simulink model "Quadrotor_Controller"  (R2019a)
settings: Solver=ode14x  StartTime=0.0  StopTime=10  FixedStep=1/100  RelTol=1e-3  EnableMultiTasking=on
undefined symbols (not defined in the file): Ap, cd, dfod, DiscIntNeverNeededParam, ioKd, ioKi, ioKp, Kd, Kp, kt, L, Newton, Pitch_0, Raphson, rho, Roll_0, Rp, X, Y, Z
libraries: sm_lib x122, fl_ps_legacy_lib x41, fl_lib x28, nesl_utility x14, sharedtransform x12, simulink x5, Electrical_Library x4, Mechanical_Library x4
(part 4 of 5)

== system Quadrotor_Controller/Quadrotor Mechanics/HUB_1_RIGID ==
  ReferenceFrame : sm_lib/Frames and Transforms/Reference Frame
  Solid : sm_lib/Body Elements/Solid  InertiaType=Custom  Mass=0.0035073100000000005  MassUnits=kg  CenterOfMass=[0.0036894251968503933 0.014803307086614171 -0.020664488188976374]  CenterOfMassUnits=in  MomentsOfInertia=[0.001075372000744001 0.0010304544609089214 0.0019974579949159888]  MomentsOfInertiaUnits=kg*in^2  ProductsOfInertia=[-1.7442184884369763e-05 2.6471572943145881e-07 3.2888585777171548e-06]  ProductsOfInertiaUnits=kg*in^2  BasedOnType=Density  Density=1000  DensityUnits=kg/(m^3)  DoExposeReferenceFrame=on  SerializedFrames=<Frames/>  GraphicType=FromGeometry  MarkerShape=Sphere  MarkerSize=10  MarkerSizeUnits=m  GraphicVisPropType=SimpleVisualProperties  GraphicDiffuseColor=[0.792157 0.819608 0.933333]  GraphicSpecularColor=[0.5 0.5 0.5 1.0]  GraphicAmbientColor=[0.15 0.15 0.15 1.0]  GraphicEmissiveColor=[0.0 0.0 0.0 1.0]  GraphicShininess=75  GraphicOpacity=1  GeometryShape=FromFile  RectangleSize=[1 1]  RectangleSizeUnits=m  BrickDimensions=[1 1 1]  BrickDimensionUnits=m  CylinderRadius=1  CylinderRadiusUnits=m  CylinderLength=1  CylinderLengthUnits=m  SphereRadius=1  SphereRadiusUnits=m  EllipsoidRadii=[1 1 1]  EllipsoidRadiiUnits=m  ExtrusionCrossSection=[1 1; -1 1; -1 -1; 1 -1]  ExtrusionCrossSectionUnits=m  ExtrusionLength=1  ExtrusionLengthUnits=m  PolygonNumSides=3  PolygonOuterRadius=1  PolygonOuterRadiusUnits=m  ExtGeomFileType=STL  ExtGeomFileName=HUB_Default_sldprt.STL  ExtGeomFileUnits=in  RevolutionCrossSection=[1 1; 1 -1; 2 -1; 2 1]  RevolutionCrossSectionUnits=m  RevolutionExtent=Full  RevolutionAngle=180  RevolutionAngleUnits=deg
  F : PMIOPort  Side=Left
  connections:
  Solid/RConn1 -- ReferenceFrame/RConn1 -- F/RConn1

== system Quadrotor_Controller/Subsystem/Triggered Subsystem ==
  In1 : Inport
  Trigger : TriggerPort  VariantControl=Variant
  Out1 : Outport
  wires:
  In1/1 -> Out1/1

== system Quadrotor_Controller/Controller/FOPD/Fractional DD ==
  In1 : Inport
  Discrete Transfer Fcn : DiscreteTransferFcn  Commented=on  Numerator=num  Denominator=den  SampleTime=Ts
  Rate Transition : RateTransition  OutPortSampleTime=Ts
  Rate Transition1 : RateTransition  OutPortSampleTime=0.01
  Transfer Fcn : TransferFcn  Numerator=num  Denominator=den
  Out1 : Outport
  wires:
  Transfer Fcn/1 -> Rate Transition1/1
  In1/1 -> Rate Transition/1
  Rate Transition/1 -> Transfer Fcn/1
  Rate Transition1/1 -> Out1/1

== system Quadrotor_Controller/Controller/FOPD GNCC IRID/Fractional DD ==
  In1 : Inport
  Discrete Transfer Fcn : DiscreteTransferFcn  Commented=on  Numerator=num  Denominator=den  SampleTime=Ts
  Rate Transition : RateTransition  OutPortSampleTime=Ts
  Rate Transition1 : RateTransition  OutPortSampleTime=0.01
  Transfer Fcn : TransferFcn  Numerator=num  Denominator=den
  Out1 : Outport
  wires:
  Transfer Fcn/1 -> Rate Transition1/1
  In1/1 -> Rate Transition/1
  Rate Transition/1 -> Transfer Fcn/1
  Rate Transition1/1 -> Out1/1

== system Quadrotor_Controller/Controller/FOPI- GNCC IRID/Fractional DD ==
  In1 : Inport
  Discrete Transfer Fcn : DiscreteTransferFcn  Commented=on  Numerator=num  Denominator=den  SampleTime=Ts
  Rate Transition : RateTransition  OutPortSampleTime=Ts
  Rate Transition1 : RateTransition  OutPortSampleTime=0.01
  Transfer Fcn : TransferFcn  Numerator=num  Denominator=den
  Out1 : Outport
  wires:
  Transfer Fcn/1 -> Rate Transition1/1
  In1/1 -> Rate Transition/1
  Rate Transition/1 -> Transfer Fcn/1
  Rate Transition1/1 -> Out1/1

== system Quadrotor_Controller/Controller/FOPID/Fractional DD ==
  In1 : Inport
  Discrete Transfer Fcn : DiscreteTransferFcn  Commented=on  Numerator=num  Denominator=den  SampleTime=Ts
  Rate Transition : RateTransition  OutPortSampleTime=Ts
  Rate Transition1 : RateTransition  OutPortSampleTime=0.01
  Transfer Fcn : TransferFcn  Numerator=num  Denominator=den
  Out1 : Outport
  wires:
  Transfer Fcn/1 -> Rate Transition1/1
  In1/1 -> Rate Transition/1
  Rate Transition/1 -> Transfer Fcn/1
  Rate Transition1/1 -> Out1/1

== system Quadrotor_Controller/Controller/FOPID/Fractional DD1 ==
  In1 : Inport
  Discrete Transfer Fcn : DiscreteTransferFcn  Commented=on  Numerator=num  Denominator=den  SampleTime=Ts
  Rate Transition : RateTransition  OutPortSampleTime=Ts
  Rate Transition1 : RateTransition  OutPortSampleTime=0.01
  Transfer Fcn : TransferFcn  Numerator=num  Denominator=den
  Out1 : Outport
  wires:
  Transfer Fcn/1 -> Rate Transition1/1
  In1/1 -> Rate Transition/1
  Rate Transition/1 -> Transfer Fcn/1
  Rate Transition1/1 -> Out1/1

== system Quadrotor_Controller/Ground Stop/FloorStop1/Translational Simscape Intf1 ==
  Ideal Force Sensor : fl_lib/Mechanical/Mechanical Sensors/Ideal Force Sensor
  Ideal Translational Velocity Source : fl_lib/Mechanical/Mechanical Sources/Ideal Translational Velocity Source
  V : PMIOPort  Side=Left
  F : PMIOPort  Port=2  Side=Right
  R : PMIOPort  Port=3  Side=Left
  C : PMIOPort  Port=4  Side=Right
  connections:
  V/RConn1 -- Ideal Translational Velocity Source/RConn1
  F/RConn1 -- Ideal Force Sensor/RConn2
  Ideal Force Sensor/LConn1 -- Ideal Translational Velocity Source/RConn2
  R/RConn1 -- Ideal Translational Velocity Source/LConn1
  Ideal Force Sensor/RConn1 -- C/RConn1

== system Quadrotor_Controller/Ground Stop/FloorStop2/Translational Simscape Intf1 ==
  Ideal Force Sensor : fl_lib/Mechanical/Mechanical Sensors/Ideal Force Sensor
  Ideal Translational Velocity Source : fl_lib/Mechanical/Mechanical Sources/Ideal Translational Velocity Source
  V : PMIOPort  Side=Left
  F : PMIOPort  Port=2  Side=Right
  R : PMIOPort  Port=3  Side=Left
  C : PMIOPort  Port=4  Side=Right
  connections:
  Ideal Force Sensor/RConn1 -- C/RConn1
  R/RConn1 -- Ideal Translational Velocity Source/LConn1
  Ideal Force Sensor/LConn1 -- Ideal Translational Velocity Source/RConn2
  F/RConn1 -- Ideal Force Sensor/RConn2
  V/RConn1 -- Ideal Translational Velocity Source/RConn1

== system Quadrotor_Controller/Ground Stop/FloorStop3/Translational Simscape Intf1 ==
  Ideal Force Sensor : fl_lib/Mechanical/Mechanical Sensors/Ideal Force Sensor
  Ideal Translational Velocity Source : fl_lib/Mechanical/Mechanical Sources/Ideal Translational Velocity Source
  V : PMIOPort  Side=Left
  F : PMIOPort  Port=2  Side=Right
  R : PMIOPort  Port=3  Side=Left
  C : PMIOPort  Port=4  Side=Right
  connections:
  Ideal Force Sensor/RConn1 -- C/RConn1
  R/RConn1 -- Ideal Translational Velocity Source/LConn1
  Ideal Force Sensor/LConn1 -- Ideal Translational Velocity Source/RConn2
  F/RConn1 -- Ideal Force Sensor/RConn2
  V/RConn1 -- Ideal Translational Velocity Source/RConn1

== system Quadrotor_Controller/Ground Stop/FloorStop4/Translational Simscape Intf1 ==
  Ideal Force Sensor : fl_lib/Mechanical/Mechanical Sensors/Ideal Force Sensor
  Ideal Translational Velocity Source : fl_lib/Mechanical/Mechanical Sources/Ideal Translational Velocity Source
  V : PMIOPort  Side=Left
  F : PMIOPort  Port=2  Side=Right
  R : PMIOPort  Port=3  Side=Left
  C : PMIOPort  Port=4  Side=Right
  connections:
  Ideal Force Sensor/RConn1 -- C/RConn1
  R/RConn1 -- Ideal Translational Velocity Source/LConn1
  Ideal Force Sensor/LConn1 -- Ideal Translational Velocity Source/RConn2
  F/RConn1 -- Ideal Force Sensor/RConn2
  V/RConn1 -- Ideal Translational Velocity Source/RConn1

== system Quadrotor_Controller/Measurements/Bus Mapping/Subsystem ==
  DCM : Inport
  AxisRotDefault : sharedtransform/Direction Cosine Matrix to Rotation Angles/AxisRotDefault  SystemSampleTime=-1
      settings: SourceProductName=Aerospace Blockset  SourceProductBaseCode=AE
  AxisRotZeroR3 : sharedtransform/Direction Cosine Matrix to Rotation Angles/AxisRotZeroR3  SystemSampleTime=-1
      settings: SourceProductName=Aerospace Blockset  SourceProductBaseCode=AE
  Get DCM Values : sharedtransform/Direction Cosine Matrix to Rotation Angles/Get DCM Values  SystemSampleTime=-1
      settings: SourceProductName=Aerospace Blockset  SourceProductBaseCode=AE
  If : If  IfExpression=(u1>=1)|(u1<=-1)
  Merge : Merge
  Selector4 : Selector  InputPortWidth=7  IndexOptions=Index vector (dialog)  Indices=3  OutputSizes=1
  Out1 : Outport
  wires:
  Merge/1 -> Out1/1
  If/1 -> AxisRotZeroR3/Action
  Selector4/1 -> If/1  "r21"
  DCM/1 -> Get DCM Values/1
  Get DCM Values/1 -> Selector4/1, AxisRotZeroR3/1, AxisRotDefault/1
  AxisRotDefault/1 -> Merge/2
  AxisRotZeroR3/1 -> Merge/1
  If/2 -> AxisRotDefault/Action

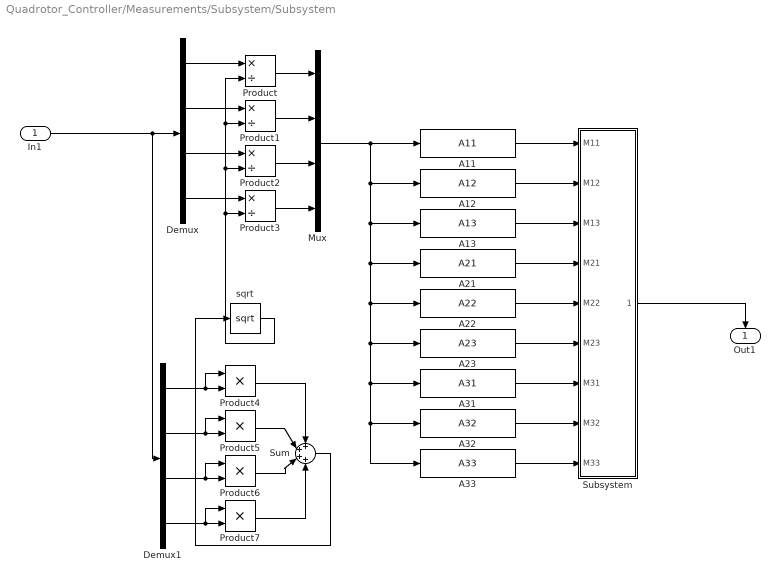
== system Quadrotor_Controller/Measurements/Subsystem/Subsystem ==
  In1 : Inport
  A11 : sharedtransform/Quaternions to  Direction Cosine Matrix/A11  SystemSampleTime=-1
      settings: SourceProductName=Aerospace Blockset  SourceProductBaseCode=AE
  A12 : sharedtransform/Quaternions to  Direction Cosine Matrix/A12  SystemSampleTime=-1
      settings: SourceProductName=Aerospace Blockset  SourceProductBaseCode=AE
  A13 : sharedtransform/Quaternions to  Direction Cosine Matrix/A13  SystemSampleTime=-1
      settings: SourceProductName=Aerospace Blockset  SourceProductBaseCode=AE
  A21 : sharedtransform/Quaternions to  Direction Cosine Matrix/A21  SystemSampleTime=-1
      settings: SourceProductName=Aerospace Blockset  SourceProductBaseCode=AE
  A22 : sharedtransform/Quaternions to  Direction Cosine Matrix/A22  SystemSampleTime=-1
      settings: SourceProductName=Aerospace Blockset  SourceProductBaseCode=AE
  A23 : sharedtransform/Quaternions to  Direction Cosine Matrix/A23  SystemSampleTime=-1
      settings: SourceProductName=Aerospace Blockset  SourceProductBaseCode=AE
  A31 : sharedtransform/Quaternions to  Direction Cosine Matrix/A31  SystemSampleTime=-1
      settings: SourceProductName=Aerospace Blockset  SourceProductBaseCode=AE
  A32 : sharedtransform/Quaternions to  Direction Cosine Matrix/A32  SystemSampleTime=-1
      settings: SourceProductName=Aerospace Blockset  SourceProductBaseCode=AE
  A33 : sharedtransform/Quaternions to  Direction Cosine Matrix/A33  SystemSampleTime=-1
      settings: SourceProductName=Aerospace Blockset  SourceProductBaseCode=AE
  Demux : Demux
  Demux1 : Demux
  Mux : Mux
  Product{,1..3} (4 alike) : Product  Inputs=*/
  Product{4..7} (4 alike) : Product
  Subsystem : Subsystem
  Sum : Sum  Inputs=4
  sqrt : Sqrt  AlgorithmType=Newton-Raphson  SaturateOnIntegerOverflow=on
  Out1 : Outport
  wires:
  Subsystem/1(Matrix) -> Out1/1
  Demux1/4 -> Product7/1, Product7/2
  Demux1/3 -> Product6/1, Product6/2
  A32/1 -> Subsystem/8(M32)
  A31/1 -> Subsystem/7(M31)
  Product5/1 -> Sum/2
  A23/1 -> Subsystem/6(M23)
  A11/1 -> Subsystem/1(M11)
  Product7/1 -> Sum/4
  Mux/1 -> A11/1, A12/1, A13/1, A21/1, A22/1, A23/1, A31/1, A32/1, A33/1
  Sum/1 -> sqrt/1
  A13/1 -> Subsystem/3(M13)
  In1/1 -> Demux1/1, Demux/1
  A21/1 -> Subsystem/4(M21)
  A12/1 -> Subsystem/2(M12)
  A22/1 -> Subsystem/5(M22)
  Demux1/2 -> Product5/1, Product5/2
  Product1/1 -> Mux/2
  A33/1 -> Subsystem/9(M33)
  sqrt/1 -> Product3/2, Product2/2, Product/2, Product1/2
  Product6/1 -> Sum/3
  Product3/1 -> Mux/4
  Demux1/1 -> Product4/1, Product4/2
  Product2/1 -> Mux/3
  Product4/1 -> Sum/1
  Demux/4 -> Product3/1
  Demux/3 -> Product2/1
  Demux/2 -> Product1/1
  Product/1 -> Mux/1
  Demux/1 -> Product/1

== system Quadrotor_Controller/Quadrotor Mechanics/ASSY_ROTOR_END_1_RIGID/CARRIER_1_RIGID ==
  ReferenceFrame : sm_lib/Frames and Transforms/Reference Frame
  Solid : sm_lib/Body Elements/Solid  InertiaType=Custom  Mass=0.0014790700000000001  MassUnits=kg  CenterOfMass=[-0.033237795275590544 -9.7131496062992118e-06 -0.051876377952755896]  CenterOfMassUnits=in  MomentsOfInertia=[0.00042507905015810019 0.00049308543617087219 0.00028994512989025968]  MomentsOfInertiaUnits=kg*in^2  ProductsOfInertia=[-6.2859755719511414e-09 -0.00014201965403930802 9.3946617893235753e-09]  ProductsOfInertiaUnits=kg*in^2  BasedOnType=Density  Density=1000  DensityUnits=kg/(m^3)  DoExposeReferenceFrame=on  SerializedFrames=<Frames/>  GraphicType=FromGeometry  MarkerShape=Sphere  MarkerSize=10  MarkerSizeUnits=m  GraphicVisPropType=SimpleVisualProperties  GraphicDiffuseColor=[0.792157 0.819608 0.933333]  GraphicSpecularColor=[0.5 0.5 0.5 1.0]  GraphicAmbientColor=[0.15 0.15 0.15 1.0]  GraphicEmissiveColor=[0.0 0.0 0.0 1.0]  GraphicShininess=75  GraphicOpacity=1  GeometryShape=FromFile  RectangleSize=[1 1]  RectangleSizeUnits=m  BrickDimensions=[1 1 1]  BrickDimensionUnits=m  CylinderRadius=1  CylinderRadiusUnits=m  CylinderLength=1  CylinderLengthUnits=m  SphereRadius=1  SphereRadiusUnits=m  EllipsoidRadii=[1 1 1]  EllipsoidRadiiUnits=m  ExtrusionCrossSection=[1 1; -1 1; -1 -1; 1 -1]  ExtrusionCrossSectionUnits=m  ExtrusionLength=1  ExtrusionLengthUnits=m  PolygonNumSides=3  PolygonOuterRadius=1  PolygonOuterRadiusUnits=m  ExtGeomFileType=STL  ExtGeomFileName=CARRIER_Default_sldprt.STL  ExtGeomFileUnits=in  RevolutionCrossSection=[1 1; 1 -1; 2 -1; 2 1]  RevolutionCrossSectionUnits=m  RevolutionExtent=Full  RevolutionAngle=180  RevolutionAngleUnits=deg
  F : PMIOPort  Side=Left
  connections:
  F/RConn1 -- ReferenceFrame/RConn1 -- Solid/RConn1

== system Quadrotor_Controller/Quadrotor Mechanics/ASSY_ROTOR_END_1_RIGID/GEAR_1_RIGID ==
  ReferenceFrame : sm_lib/Frames and Transforms/Reference Frame
  Solid : sm_lib/Body Elements/Solid  InertiaType=Custom  Mass=0.00036074399999999997  MassUnits=kg  CenterOfMass=[7.4797244094488169e-08 0.00011347952755905511 0.0055607480314960617]  CenterOfMassUnits=in  MomentsOfInertia=[1.348894847789695e-05 1.3494962489924976e-05 2.6179087358174708e-05]  MomentsOfInertiaUnits=kg*in^2  ProductsOfInertia=[3.0075950151900291e-09 8.3272366544733066e-13 -5.1715698431396846e-12]  ProductsOfInertiaUnits=kg*in^2  BasedOnType=Density  Density=1000  DensityUnits=kg/(m^3)  DoExposeReferenceFrame=on  SerializedFrames=<Frames/>  GraphicType=FromGeometry  MarkerShape=Sphere  MarkerSize=10  MarkerSizeUnits=m  GraphicVisPropType=SimpleVisualProperties  GraphicDiffuseColor=[0.792157 0.819608 0.933333]  GraphicSpecularColor=[0.5 0.5 0.5 1.0]  GraphicAmbientColor=[0.15 0.15 0.15 1.0]  GraphicEmissiveColor=[0.0 0.0 0.0 1.0]  GraphicShininess=75  GraphicOpacity=1  GeometryShape=FromFile  RectangleSize=[1 1]  RectangleSizeUnits=m  BrickDimensions=[1 1 1]  BrickDimensionUnits=m  CylinderRadius=1  CylinderRadiusUnits=m  CylinderLength=1  CylinderLengthUnits=m  SphereRadius=1  SphereRadiusUnits=m  EllipsoidRadii=[1 1 1]  EllipsoidRadiiUnits=m  ExtrusionCrossSection=[1 1; -1 1; -1 -1; 1 -1]  ExtrusionCrossSectionUnits=m  ExtrusionLength=1  ExtrusionLengthUnits=m  PolygonNumSides=3  PolygonOuterRadius=1  PolygonOuterRadiusUnits=m  ExtGeomFileType=STL  ExtGeomFileName=GEAR_Default_sldprt.STL  ExtGeomFileUnits=in  RevolutionCrossSection=[1 1; 1 -1; 2 -1; 2 1]  RevolutionCrossSectionUnits=m  RevolutionExtent=Full  RevolutionAngle=180  RevolutionAngleUnits=deg
  F : PMIOPort  Side=Left
  connections:
  F/RConn1 -- ReferenceFrame/RConn1 -- Solid/RConn1

== system Quadrotor_Controller/Quadrotor Mechanics/ASSY_ROTOR_END_1_RIGID/MOTOR_1_RIGID ==
  ReferenceFrame : sm_lib/Frames and Transforms/Reference Frame
  Solid : sm_lib/Body Elements/Solid  InertiaType=Custom  Mass=0.0011134299999999999  MassUnits=kg  CenterOfMass=[0 0 -0.39208425196850388]  CenterOfMassUnits=in  MomentsOfInertia=[6.765593031186059e-05 6.765593031186059e-05 1.5113894227788452e-05]  MomentsOfInertiaUnits=kg*in^2  ProductsOfInertia=[0 0 0]  ProductsOfInertiaUnits=kg*in^2  BasedOnType=Density  Density=1000  DensityUnits=kg/(m^3)  DoExposeReferenceFrame=on  SerializedFrames=<Frames/>  GraphicType=FromGeometry  MarkerShape=Sphere  MarkerSize=10  MarkerSizeUnits=m  GraphicVisPropType=SimpleVisualProperties  GraphicDiffuseColor=[0.792157 0.819608 0.933333]  GraphicSpecularColor=[0.5 0.5 0.5 1.0]  GraphicAmbientColor=[0.15 0.15 0.15 1.0]  GraphicEmissiveColor=[0.0 0.0 0.0 1.0]  GraphicShininess=75  GraphicOpacity=1  GeometryShape=FromFile  RectangleSize=[1 1]  RectangleSizeUnits=m  BrickDimensions=[1 1 1]  BrickDimensionUnits=m  CylinderRadius=1  CylinderRadiusUnits=m  CylinderLength=1  CylinderLengthUnits=m  SphereRadius=1  SphereRadiusUnits=m  EllipsoidRadii=[1 1 1]  EllipsoidRadiiUnits=m  ExtrusionCrossSection=[1 1; -1 1; -1 -1; 1 -1]  ExtrusionCrossSectionUnits=m  ExtrusionLength=1  ExtrusionLengthUnits=m  PolygonNumSides=3  PolygonOuterRadius=1  PolygonOuterRadiusUnits=m  ExtGeomFileType=STL  ExtGeomFileName=MOTOR_Default_sldprt.STL  ExtGeomFileUnits=in  RevolutionCrossSection=[1 1; 1 -1; 2 -1; 2 1]  RevolutionCrossSectionUnits=m  RevolutionExtent=Full  RevolutionAngle=180  RevolutionAngleUnits=deg
  F : PMIOPort  Side=Left
  connections:
  F/RConn1 -- ReferenceFrame/RConn1 -- Solid/RConn1

== system Quadrotor_Controller/Quadrotor Mechanics/ASSY_ROTOR_END_1_RIGID/ROTOR_1_RIGID ==
  ReferenceFrame : sm_lib/Frames and Transforms/Reference Frame
  Solid : sm_lib/Body Elements/Solid  InertiaType=Custom  Mass=0.00139186  MassUnits=kg  CenterOfMass=[-3.0265944881889758e-07 -1.0311377952755904e-07 0.46932283464566926]  CenterOfMassUnits=in  MomentsOfInertia=[4.152148304296607e-05 0.0024363103726207443 0.0024351323702647395]  MomentsOfInertiaUnits=kg*in^2  ProductsOfInertia=[-1.4486886973773942e-11 3.7024769049538088e-11 -4.6396242792485567e-05]  ProductsOfInertiaUnits=kg*in^2  BasedOnType=Density  Density=1000  DensityUnits=kg/(m^3)  DoExposeReferenceFrame=on  SerializedFrames=<Frames/>  GraphicType=FromGeometry  MarkerShape=Sphere  MarkerSize=10  MarkerSizeUnits=m  GraphicVisPropType=SimpleVisualProperties  GraphicDiffuseColor=[0.792157 0.819608 0.933333]  GraphicSpecularColor=[0.5 0.5 0.5 1.0]  GraphicAmbientColor=[0.15 0.15 0.15 1.0]  GraphicEmissiveColor=[0.0 0.0 0.0 1.0]  GraphicShininess=75  GraphicOpacity=1  GeometryShape=FromFile  RectangleSize=[1 1]  RectangleSizeUnits=m  BrickDimensions=[1 1 1]  BrickDimensionUnits=m  CylinderRadius=1  CylinderRadiusUnits=m  CylinderLength=1  CylinderLengthUnits=m  SphereRadius=1  SphereRadiusUnits=m  EllipsoidRadii=[1 1 1]  EllipsoidRadiiUnits=m  ExtrusionCrossSection=[1 1; -1 1; -1 -1; 1 -1]  ExtrusionCrossSectionUnits=m  ExtrusionLength=1  ExtrusionLengthUnits=m  PolygonNumSides=3  PolygonOuterRadius=1  PolygonOuterRadiusUnits=m  ExtGeomFileType=STL  ExtGeomFileName=ROTOR_Default_sldprt.STL  ExtGeomFileUnits=in  RevolutionCrossSection=[1 1; 1 -1; 2 -1; 2 1]  RevolutionCrossSectionUnits=m  RevolutionExtent=Full  RevolutionAngle=180  RevolutionAngleUnits=deg
  F : PMIOPort  Side=Left
  connections:
  F/RConn1 -- ReferenceFrame/RConn1 -- Solid/RConn1

== system Quadrotor_Controller/Quadrotor Mechanics/ASSY_ROTOR_END_1_RIGID/SHAFT_1_RIGID ==
  ReferenceFrame : sm_lib/Frames and Transforms/Reference Frame
  Solid : sm_lib/Body Elements/Solid  InertiaType=Custom  Mass=0.00027398899999999998  MassUnits=kg  CenterOfMass=[0.75914960629921258 0 0.00073037401574803135]  CenterOfMassUnits=in  MomentsOfInertia=[4.8873147746295477e-07 5.0754386508772994e-05 5.076306652613304e-05]  MomentsOfInertiaUnits=kg*in^2  ProductsOfInertia=[0 -1.2690278380556758e-07 0]  ProductsOfInertiaUnits=kg*in^2  BasedOnType=Density  Density=1000  DensityUnits=kg/(m^3)  DoExposeReferenceFrame=on  SerializedFrames=<Frames/>  GraphicType=FromGeometry  MarkerShape=Sphere  MarkerSize=10  MarkerSizeUnits=m  GraphicVisPropType=SimpleVisualProperties  GraphicDiffuseColor=[0.792157 0.819608 0.933333]  GraphicSpecularColor=[0.5 0.5 0.5 1.0]  GraphicAmbientColor=[0.15 0.15 0.15 1.0]  GraphicEmissiveColor=[0.0 0.0 0.0 1.0]  GraphicShininess=75  GraphicOpacity=1  GeometryShape=FromFile  RectangleSize=[1 1]  RectangleSizeUnits=m  BrickDimensions=[1 1 1]  BrickDimensionUnits=m  CylinderRadius=1  CylinderRadiusUnits=m  CylinderLength=1  CylinderLengthUnits=m  SphereRadius=1  SphereRadiusUnits=m  EllipsoidRadii=[1 1 1]  EllipsoidRadiiUnits=m  ExtrusionCrossSection=[1 1; -1 1; -1 -1; 1 -1]  ExtrusionCrossSectionUnits=m  ExtrusionLength=1  ExtrusionLengthUnits=m  PolygonNumSides=3  PolygonOuterRadius=1  PolygonOuterRadiusUnits=m  ExtGeomFileType=STL  ExtGeomFileName=SHAFT_Default_sldprt.STL  ExtGeomFileUnits=in  RevolutionCrossSection=[1 1; 1 -1; 2 -1; 2 1]  RevolutionCrossSectionUnits=m  RevolutionExtent=Full  RevolutionAngle=180  RevolutionAngleUnits=deg
  F : PMIOPort  Side=Left
  connections:
  F/RConn1 -- ReferenceFrame/RConn1 -- Solid/RConn1

== system Quadrotor_Controller/Quadrotor Mechanics/ASSY_ROTOR_END_1_RIGID/TUBE_1_RIGID ==
  ReferenceFrame : sm_lib/Frames and Transforms/Reference Frame
  Solid : sm_lib/Body Elements/Solid  InertiaType=Custom  Mass=0.00058215999999999997  MassUnits=kg  CenterOfMass=[1.6249999999999998 0 0]  CenterOfMassUnits=in  MomentsOfInertia=[1.6501023002045999e-06 0.00051324787649575281 0.00051324787649575281]  MomentsOfInertiaUnits=kg*in^2  ProductsOfInertia=[0 0 0]  ProductsOfInertiaUnits=kg*in^2  BasedOnType=Density  Density=1000  DensityUnits=kg/(m^3)  DoExposeReferenceFrame=on  SerializedFrames=<Frames/>  GraphicType=FromGeometry  MarkerShape=Sphere  MarkerSize=10  MarkerSizeUnits=m  GraphicVisPropType=SimpleVisualProperties  GraphicDiffuseColor=[0.792157 0.819608 0.933333]  GraphicSpecularColor=[0.5 0.5 0.5 1.0]  GraphicAmbientColor=[0.15 0.15 0.15 1.0]  GraphicEmissiveColor=[0.0 0.0 0.0 1.0]  GraphicShininess=75  GraphicOpacity=1  GeometryShape=FromFile  RectangleSize=[1 1]  RectangleSizeUnits=m  BrickDimensions=[1 1 1]  BrickDimensionUnits=m  CylinderRadius=1  CylinderRadiusUnits=m  CylinderLength=1  CylinderLengthUnits=m  SphereRadius=1  SphereRadiusUnits=m  EllipsoidRadii=[1 1 1]  EllipsoidRadiiUnits=m  ExtrusionCrossSection=[1 1; -1 1; -1 -1; 1 -1]  ExtrusionCrossSectionUnits=m  ExtrusionLength=1  ExtrusionLengthUnits=m  PolygonNumSides=3  PolygonOuterRadius=1  PolygonOuterRadiusUnits=m  ExtGeomFileType=STL  ExtGeomFileName=TUBE_Default_sldprt.STL  ExtGeomFileUnits=in  RevolutionCrossSection=[1 1; 1 -1; 2 -1; 2 1]  RevolutionCrossSectionUnits=m  RevolutionExtent=Full  RevolutionAngle=180  RevolutionAngleUnits=deg
  F : PMIOPort  Side=Left
  connections:
  F/RConn1 -- ReferenceFrame/RConn1 -- Solid/RConn1

== system Quadrotor_Controller/Quadrotor Mechanics/ASSY_ROTOR_END_1_RIGID/TUBE_END_1_RIGID ==
  ReferenceFrame : sm_lib/Frames and Transforms/Reference Frame
  Solid : sm_lib/Body Elements/Solid  InertiaType=Custom  Mass=0.0014182299999999999  MassUnits=kg  CenterOfMass=[-0.0069902755905511807 -0.030264921259842512 0.077340944881889764]  CenterOfMassUnits=in  MomentsOfInertia=[0.00018641422282844559 0.00010295260090520178 0.00012412114824229644]  MomentsOfInertiaUnits=kg*in^2  ProductsOfInertia=[-4.6923243846487677e-05 7.0815766631533238e-07 1.3636989273978543e-06]  ProductsOfInertiaUnits=kg*in^2  BasedOnType=Density  Density=1000  DensityUnits=kg/(m^3)  DoExposeReferenceFrame=on  SerializedFrames=<Frames/>  GraphicType=FromGeometry  MarkerShape=Sphere  MarkerSize=10  MarkerSizeUnits=m  GraphicVisPropType=SimpleVisualProperties  GraphicDiffuseColor=[0.792157 0.819608 0.933333]  GraphicSpecularColor=[0.5 0.5 0.5 1.0]  GraphicAmbientColor=[0.15 0.15 0.15 1.0]  GraphicEmissiveColor=[0.0 0.0 0.0 1.0]  GraphicShininess=75  GraphicOpacity=1  GeometryShape=FromFile  RectangleSize=[1 1]  RectangleSizeUnits=m  BrickDimensions=[1 1 1]  BrickDimensionUnits=m  CylinderRadius=1  CylinderRadiusUnits=m  CylinderLength=1  CylinderLengthUnits=m  SphereRadius=1  SphereRadiusUnits=m  EllipsoidRadii=[1 1 1]  EllipsoidRadiiUnits=m  ExtrusionCrossSection=[1 1; -1 1; -1 -1; 1 -1]  ExtrusionCrossSectionUnits=m  ExtrusionLength=1  ExtrusionLengthUnits=m  PolygonNumSides=3  PolygonOuterRadius=1  PolygonOuterRadiusUnits=m  ExtGeomFileType=STL  ExtGeomFileName=TUBE END_Default_sldprt.STL  ExtGeomFileUnits=in  RevolutionCrossSection=[1 1; 1 -1; 2 -1; 2 1]  RevolutionCrossSectionUnits=m  RevolutionExtent=Full  RevolutionAngle=180  RevolutionAngleUnits=deg
  F : PMIOPort  Side=Left
  connections:
  F/RConn1 -- ReferenceFrame/RConn1 -- Solid/RConn1

== system Quadrotor_Controller/Quadrotor Mechanics/ASSY_ROTOR_END_2_RIGID/CARRIER_1_RIGID ==
  ReferenceFrame : sm_lib/Frames and Transforms/Reference Frame
  Solid : sm_lib/Body Elements/Solid  InertiaType=Custom  Mass=0.0014790700000000001  MassUnits=kg  CenterOfMass=[-0.033237795275590544 -9.7131496062992118e-06 -0.051876377952755896]  CenterOfMassUnits=in  MomentsOfInertia=[0.00042507905015810019 0.00049308543617087219 0.00028994512989025968]  MomentsOfInertiaUnits=kg*in^2  ProductsOfInertia=[-6.2859755719511414e-09 -0.00014201965403930802 9.3946617893235753e-09]  ProductsOfInertiaUnits=kg*in^2  BasedOnType=Density  Density=1000  DensityUnits=kg/(m^3)  DoExposeReferenceFrame=on  SerializedFrames=<Frames/>  GraphicType=FromGeometry  MarkerShape=Sphere  MarkerSize=10  MarkerSizeUnits=m  GraphicVisPropType=SimpleVisualProperties  GraphicDiffuseColor=[0.792157 0.819608 0.933333]  GraphicSpecularColor=[0.5 0.5 0.5 1.0]  GraphicAmbientColor=[0.15 0.15 0.15 1.0]  GraphicEmissiveColor=[0.0 0.0 0.0 1.0]  GraphicShininess=75  GraphicOpacity=1  GeometryShape=FromFile  RectangleSize=[1 1]  RectangleSizeUnits=m  BrickDimensions=[1 1 1]  BrickDimensionUnits=m  CylinderRadius=1  CylinderRadiusUnits=m  CylinderLength=1  CylinderLengthUnits=m  SphereRadius=1  SphereRadiusUnits=m  EllipsoidRadii=[1 1 1]  EllipsoidRadiiUnits=m  ExtrusionCrossSection=[1 1; -1 1; -1 -1; 1 -1]  ExtrusionCrossSectionUnits=m  ExtrusionLength=1  ExtrusionLengthUnits=m  PolygonNumSides=3  PolygonOuterRadius=1  PolygonOuterRadiusUnits=m  ExtGeomFileType=STL  ExtGeomFileName=CARRIER_Default_sldprt.STL  ExtGeomFileUnits=in  RevolutionCrossSection=[1 1; 1 -1; 2 -1; 2 1]  RevolutionCrossSectionUnits=m  RevolutionExtent=Full  RevolutionAngle=180  RevolutionAngleUnits=deg
  F : PMIOPort  Side=Left
  connections:
  F/RConn1 -- ReferenceFrame/RConn1 -- Solid/RConn1

== system Quadrotor_Controller/Quadrotor Mechanics/ASSY_ROTOR_END_2_RIGID/GEAR_1_RIGID ==
  ReferenceFrame : sm_lib/Frames and Transforms/Reference Frame
  Solid : sm_lib/Body Elements/Solid  InertiaType=Custom  Mass=0.00036074399999999997  MassUnits=kg  CenterOfMass=[7.4797244094488169e-08 0.00011347952755905511 0.0055607480314960617]  CenterOfMassUnits=in  MomentsOfInertia=[1.348894847789695e-05 1.3494962489924976e-05 2.6179087358174708e-05]  MomentsOfInertiaUnits=kg*in^2  ProductsOfInertia=[3.0075950151900291e-09 8.3272366544733066e-13 -5.1715698431396846e-12]  ProductsOfInertiaUnits=kg*in^2  BasedOnType=Density  Density=1000  DensityUnits=kg/(m^3)  DoExposeReferenceFrame=on  SerializedFrames=<Frames/>  GraphicType=FromGeometry  MarkerShape=Sphere  MarkerSize=10  MarkerSizeUnits=m  GraphicVisPropType=SimpleVisualProperties  GraphicDiffuseColor=[0.792157 0.819608 0.933333]  GraphicSpecularColor=[0.5 0.5 0.5 1.0]  GraphicAmbientColor=[0.15 0.15 0.15 1.0]  GraphicEmissiveColor=[0.0 0.0 0.0 1.0]  GraphicShininess=75  GraphicOpacity=1  GeometryShape=FromFile  RectangleSize=[1 1]  RectangleSizeUnits=m  BrickDimensions=[1 1 1]  BrickDimensionUnits=m  CylinderRadius=1  CylinderRadiusUnits=m  CylinderLength=1  CylinderLengthUnits=m  SphereRadius=1  SphereRadiusUnits=m  EllipsoidRadii=[1 1 1]  EllipsoidRadiiUnits=m  ExtrusionCrossSection=[1 1; -1 1; -1 -1; 1 -1]  ExtrusionCrossSectionUnits=m  ExtrusionLength=1  ExtrusionLengthUnits=m  PolygonNumSides=3  PolygonOuterRadius=1  PolygonOuterRadiusUnits=m  ExtGeomFileType=STL  ExtGeomFileName=GEAR_Default_sldprt.STL  ExtGeomFileUnits=in  RevolutionCrossSection=[1 1; 1 -1; 2 -1; 2 1]  RevolutionCrossSectionUnits=m  RevolutionExtent=Full  RevolutionAngle=180  RevolutionAngleUnits=deg
  F : PMIOPort  Side=Left
  connections:
  F/RConn1 -- ReferenceFrame/RConn1 -- Solid/RConn1

== system Quadrotor_Controller/Quadrotor Mechanics/ASSY_ROTOR_END_2_RIGID/MOTOR_1_RIGID ==
  ReferenceFrame : sm_lib/Frames and Transforms/Reference Frame
  Solid : sm_lib/Body Elements/Solid  InertiaType=Custom  Mass=0.0011134299999999999  MassUnits=kg  CenterOfMass=[0 0 -0.39208425196850388]  CenterOfMassUnits=in  MomentsOfInertia=[6.765593031186059e-05 6.765593031186059e-05 1.5113894227788452e-05]  MomentsOfInertiaUnits=kg*in^2  ProductsOfInertia=[0 0 0]  ProductsOfInertiaUnits=kg*in^2  BasedOnType=Density  Density=1000  DensityUnits=kg/(m^3)  DoExposeReferenceFrame=on  SerializedFrames=<Frames/>  GraphicType=FromGeometry  MarkerShape=Sphere  MarkerSize=10  MarkerSizeUnits=m  GraphicVisPropType=SimpleVisualProperties  GraphicDiffuseColor=[0.792157 0.819608 0.933333]  GraphicSpecularColor=[0.5 0.5 0.5 1.0]  GraphicAmbientColor=[0.15 0.15 0.15 1.0]  GraphicEmissiveColor=[0.0 0.0 0.0 1.0]  GraphicShininess=75  GraphicOpacity=1  GeometryShape=FromFile  RectangleSize=[1 1]  RectangleSizeUnits=m  BrickDimensions=[1 1 1]  BrickDimensionUnits=m  CylinderRadius=1  CylinderRadiusUnits=m  CylinderLength=1  CylinderLengthUnits=m  SphereRadius=1  SphereRadiusUnits=m  EllipsoidRadii=[1 1 1]  EllipsoidRadiiUnits=m  ExtrusionCrossSection=[1 1; -1 1; -1 -1; 1 -1]  ExtrusionCrossSectionUnits=m  ExtrusionLength=1  ExtrusionLengthUnits=m  PolygonNumSides=3  PolygonOuterRadius=1  PolygonOuterRadiusUnits=m  ExtGeomFileType=STL  ExtGeomFileName=MOTOR_Default_sldprt.STL  ExtGeomFileUnits=in  RevolutionCrossSection=[1 1; 1 -1; 2 -1; 2 1]  RevolutionCrossSectionUnits=m  RevolutionExtent=Full  RevolutionAngle=180  RevolutionAngleUnits=deg
  F : PMIOPort  Side=Left
  connections:
  F/RConn1 -- ReferenceFrame/RConn1 -- Solid/RConn1

== system Quadrotor_Controller/Quadrotor Mechanics/ASSY_ROTOR_END_2_RIGID/ROTOR_1_RIGID ==
  ReferenceFrame : sm_lib/Frames and Transforms/Reference Frame
  Solid : sm_lib/Body Elements/Solid  InertiaType=Custom  Mass=0.00139186  MassUnits=kg  CenterOfMass=[-3.0265944881889758e-07 -1.0311377952755904e-07 0.46932283464566926]  CenterOfMassUnits=in  MomentsOfInertia=[4.152148304296607e-05 0.0024363103726207443 0.0024351323702647395]  MomentsOfInertiaUnits=kg*in^2  ProductsOfInertia=[-1.4486886973773942e-11 3.7024769049538088e-11 -4.6396242792485567e-05]  ProductsOfInertiaUnits=kg*in^2  BasedOnType=Density  Density=1000  DensityUnits=kg/(m^3)  DoExposeReferenceFrame=on  SerializedFrames=<Frames/>  GraphicType=FromGeometry  MarkerShape=Sphere  MarkerSize=10  MarkerSizeUnits=m  GraphicVisPropType=SimpleVisualProperties  GraphicDiffuseColor=[0.792157 0.819608 0.933333]  GraphicSpecularColor=[0.5 0.5 0.5 1.0]  GraphicAmbientColor=[0.15 0.15 0.15 1.0]  GraphicEmissiveColor=[0.0 0.0 0.0 1.0]  GraphicShininess=75  GraphicOpacity=1  GeometryShape=FromFile  RectangleSize=[1 1]  RectangleSizeUnits=m  BrickDimensions=[1 1 1]  BrickDimensionUnits=m  CylinderRadius=1  CylinderRadiusUnits=m  CylinderLength=1  CylinderLengthUnits=m  SphereRadius=1  SphereRadiusUnits=m  EllipsoidRadii=[1 1 1]  EllipsoidRadiiUnits=m  ExtrusionCrossSection=[1 1; -1 1; -1 -1; 1 -1]  ExtrusionCrossSectionUnits=m  ExtrusionLength=1  ExtrusionLengthUnits=m  PolygonNumSides=3  PolygonOuterRadius=1  PolygonOuterRadiusUnits=m  ExtGeomFileType=STL  ExtGeomFileName=ROTOR_Default_sldprt.STL  ExtGeomFileUnits=in  RevolutionCrossSection=[1 1; 1 -1; 2 -1; 2 1]  RevolutionCrossSectionUnits=m  RevolutionExtent=Full  RevolutionAngle=180  RevolutionAngleUnits=deg
  F : PMIOPort  Side=Left
  connections:
  F/RConn1 -- ReferenceFrame/RConn1 -- Solid/RConn1

== system Quadrotor_Controller/Quadrotor Mechanics/ASSY_ROTOR_END_2_RIGID/SHAFT_1_RIGID ==
  ReferenceFrame : sm_lib/Frames and Transforms/Reference Frame
  Solid : sm_lib/Body Elements/Solid  InertiaType=Custom  Mass=0.00027398899999999998  MassUnits=kg  CenterOfMass=[0.75914960629921258 0 0.00073037401574803135]  CenterOfMassUnits=in  MomentsOfInertia=[4.8873147746295477e-07 5.0754386508772994e-05 5.076306652613304e-05]  MomentsOfInertiaUnits=kg*in^2  ProductsOfInertia=[0 -1.2690278380556758e-07 0]  ProductsOfInertiaUnits=kg*in^2  BasedOnType=Density  Density=1000  DensityUnits=kg/(m^3)  DoExposeReferenceFrame=on  SerializedFrames=<Frames/>  GraphicType=FromGeometry  MarkerShape=Sphere  MarkerSize=10  MarkerSizeUnits=m  GraphicVisPropType=SimpleVisualProperties  GraphicDiffuseColor=[0.792157 0.819608 0.933333]  GraphicSpecularColor=[0.5 0.5 0.5 1.0]  GraphicAmbientColor=[0.15 0.15 0.15 1.0]  GraphicEmissiveColor=[0.0 0.0 0.0 1.0]  GraphicShininess=75  GraphicOpacity=1  GeometryShape=FromFile  RectangleSize=[1 1]  RectangleSizeUnits=m  BrickDimensions=[1 1 1]  BrickDimensionUnits=m  CylinderRadius=1  CylinderRadiusUnits=m  CylinderLength=1  CylinderLengthUnits=m  SphereRadius=1  SphereRadiusUnits=m  EllipsoidRadii=[1 1 1]  EllipsoidRadiiUnits=m  ExtrusionCrossSection=[1 1; -1 1; -1 -1; 1 -1]  ExtrusionCrossSectionUnits=m  ExtrusionLength=1  ExtrusionLengthUnits=m  PolygonNumSides=3  PolygonOuterRadius=1  PolygonOuterRadiusUnits=m  ExtGeomFileType=STL  ExtGeomFileName=SHAFT_Default_sldprt.STL  ExtGeomFileUnits=in  RevolutionCrossSection=[1 1; 1 -1; 2 -1; 2 1]  RevolutionCrossSectionUnits=m  RevolutionExtent=Full  RevolutionAngle=180  RevolutionAngleUnits=deg
  F : PMIOPort  Side=Left
  connections:
  F/RConn1 -- ReferenceFrame/RConn1 -- Solid/RConn1

== system Quadrotor_Controller/Quadrotor Mechanics/ASSY_ROTOR_END_2_RIGID/TUBE_1_RIGID ==
  ReferenceFrame : sm_lib/Frames and Transforms/Reference Frame
  Solid : sm_lib/Body Elements/Solid  InertiaType=Custom  Mass=0.00058215999999999997  MassUnits=kg  CenterOfMass=[1.6249999999999998 0 0]  CenterOfMassUnits=in  MomentsOfInertia=[1.6501023002045999e-06 0.00051324787649575281 0.00051324787649575281]  MomentsOfInertiaUnits=kg*in^2  ProductsOfInertia=[0 0 0]  ProductsOfInertiaUnits=kg*in^2  BasedOnType=Density  Density=1000  DensityUnits=kg/(m^3)  DoExposeReferenceFrame=on  SerializedFrames=<Frames/>  GraphicType=FromGeometry  MarkerShape=Sphere  MarkerSize=10  MarkerSizeUnits=m  GraphicVisPropType=SimpleVisualProperties  GraphicDiffuseColor=[0.792157 0.819608 0.933333]  GraphicSpecularColor=[0.5 0.5 0.5 1.0]  GraphicAmbientColor=[0.15 0.15 0.15 1.0]  GraphicEmissiveColor=[0.0 0.0 0.0 1.0]  GraphicShininess=75  GraphicOpacity=1  GeometryShape=FromFile  RectangleSize=[1 1]  RectangleSizeUnits=m  BrickDimensions=[1 1 1]  BrickDimensionUnits=m  CylinderRadius=1  CylinderRadiusUnits=m  CylinderLength=1  CylinderLengthUnits=m  SphereRadius=1  SphereRadiusUnits=m  EllipsoidRadii=[1 1 1]  EllipsoidRadiiUnits=m  ExtrusionCrossSection=[1 1; -1 1; -1 -1; 1 -1]  ExtrusionCrossSectionUnits=m  ExtrusionLength=1  ExtrusionLengthUnits=m  PolygonNumSides=3  PolygonOuterRadius=1  PolygonOuterRadiusUnits=m  ExtGeomFileType=STL  ExtGeomFileName=TUBE_Default_sldprt.STL  ExtGeomFileUnits=in  RevolutionCrossSection=[1 1; 1 -1; 2 -1; 2 1]  RevolutionCrossSectionUnits=m  RevolutionExtent=Full  RevolutionAngle=180  RevolutionAngleUnits=deg
  F : PMIOPort  Side=Left
  connections:
  F/RConn1 -- ReferenceFrame/RConn1 -- Solid/RConn1

== system Quadrotor_Controller/Quadrotor Mechanics/ASSY_ROTOR_END_2_RIGID/TUBE_END_1_RIGID ==
  ReferenceFrame : sm_lib/Frames and Transforms/Reference Frame
  Solid : sm_lib/Body Elements/Solid  InertiaType=Custom  Mass=0.0014182299999999999  MassUnits=kg  CenterOfMass=[-0.0069902755905511807 -0.030264921259842512 0.077340944881889764]  CenterOfMassUnits=in  MomentsOfInertia=[0.00018641422282844559 0.00010295260090520178 0.00012412114824229644]  MomentsOfInertiaUnits=kg*in^2  ProductsOfInertia=[-4.6923243846487677e-05 7.0815766631533238e-07 1.3636989273978543e-06]  ProductsOfInertiaUnits=kg*in^2  BasedOnType=Density  Density=1000  DensityUnits=kg/(m^3)  DoExposeReferenceFrame=on  SerializedFrames=<Frames/>  GraphicType=FromGeometry  MarkerShape=Sphere  MarkerSize=10  MarkerSizeUnits=m  GraphicVisPropType=SimpleVisualProperties  GraphicDiffuseColor=[0.792157 0.819608 0.933333]  GraphicSpecularColor=[0.5 0.5 0.5 1.0]  GraphicAmbientColor=[0.15 0.15 0.15 1.0]  GraphicEmissiveColor=[0.0 0.0 0.0 1.0]  GraphicShininess=75  GraphicOpacity=1  GeometryShape=FromFile  RectangleSize=[1 1]  RectangleSizeUnits=m  BrickDimensions=[1 1 1]  BrickDimensionUnits=m  CylinderRadius=1  CylinderRadiusUnits=m  CylinderLength=1  CylinderLengthUnits=m  SphereRadius=1  SphereRadiusUnits=m  EllipsoidRadii=[1 1 1]  EllipsoidRadiiUnits=m  ExtrusionCrossSection=[1 1; -1 1; -1 -1; 1 -1]  ExtrusionCrossSectionUnits=m  ExtrusionLength=1  ExtrusionLengthUnits=m  PolygonNumSides=3  PolygonOuterRadius=1  PolygonOuterRadiusUnits=m  ExtGeomFileType=STL  ExtGeomFileName=TUBE END_Default_sldprt.STL  ExtGeomFileUnits=in  RevolutionCrossSection=[1 1; 1 -1; 2 -1; 2 1]  RevolutionCrossSectionUnits=m  RevolutionExtent=Full  RevolutionAngle=180  RevolutionAngleUnits=deg
  F : PMIOPort  Side=Left
  connections:
  F/RConn1 -- ReferenceFrame/RConn1 -- Solid/RConn1

== system Quadrotor_Controller/Quadrotor Mechanics/ASSY_ROTOR_END_3_RIGID/CARRIER_1_RIGID ==
  ReferenceFrame : sm_lib/Frames and Transforms/Reference Frame
  Solid : sm_lib/Body Elements/Solid  InertiaType=Custom  Mass=0.0014790700000000001  MassUnits=kg  CenterOfMass=[-0.033237795275590544 -9.7131496062992118e-06 -0.051876377952755896]  CenterOfMassUnits=in  MomentsOfInertia=[0.00042507905015810019 0.00049308543617087219 0.00028994512989025968]  MomentsOfInertiaUnits=kg*in^2  ProductsOfInertia=[-6.2859755719511414e-09 -0.00014201965403930802 9.3946617893235753e-09]  ProductsOfInertiaUnits=kg*in^2  BasedOnType=Density  Density=1000  DensityUnits=kg/(m^3)  DoExposeReferenceFrame=on  SerializedFrames=<Frames/>  GraphicType=FromGeometry  MarkerShape=Sphere  MarkerSize=10  MarkerSizeUnits=m  GraphicVisPropType=SimpleVisualProperties  GraphicDiffuseColor=[0.792157 0.819608 0.933333]  GraphicSpecularColor=[0.5 0.5 0.5 1.0]  GraphicAmbientColor=[0.15 0.15 0.15 1.0]  GraphicEmissiveColor=[0.0 0.0 0.0 1.0]  GraphicShininess=75  GraphicOpacity=1  GeometryShape=FromFile  RectangleSize=[1 1]  RectangleSizeUnits=m  BrickDimensions=[1 1 1]  BrickDimensionUnits=m  CylinderRadius=1  CylinderRadiusUnits=m  CylinderLength=1  CylinderLengthUnits=m  SphereRadius=1  SphereRadiusUnits=m  EllipsoidRadii=[1 1 1]  EllipsoidRadiiUnits=m  ExtrusionCrossSection=[1 1; -1 1; -1 -1; 1 -1]  ExtrusionCrossSectionUnits=m  ExtrusionLength=1  ExtrusionLengthUnits=m  PolygonNumSides=3  PolygonOuterRadius=1  PolygonOuterRadiusUnits=m  ExtGeomFileType=STL  ExtGeomFileName=CARRIER_Default_sldprt.STL  ExtGeomFileUnits=in  RevolutionCrossSection=[1 1; 1 -1; 2 -1; 2 1]  RevolutionCrossSectionUnits=m  RevolutionExtent=Full  RevolutionAngle=180  RevolutionAngleUnits=deg
  F : PMIOPort  Side=Left
  connections:
  F/RConn1 -- ReferenceFrame/RConn1 -- Solid/RConn1

== system Quadrotor_Controller/Quadrotor Mechanics/ASSY_ROTOR_END_3_RIGID/GEAR_1_RIGID ==
  ReferenceFrame : sm_lib/Frames and Transforms/Reference Frame
  Solid : sm_lib/Body Elements/Solid  InertiaType=Custom  Mass=0.00036074399999999997  MassUnits=kg  CenterOfMass=[7.4797244094488169e-08 0.00011347952755905511 0.0055607480314960617]  CenterOfMassUnits=in  MomentsOfInertia=[1.348894847789695e-05 1.3494962489924976e-05 2.6179087358174708e-05]  MomentsOfInertiaUnits=kg*in^2  ProductsOfInertia=[3.0075950151900291e-09 8.3272366544733066e-13 -5.1715698431396846e-12]  ProductsOfInertiaUnits=kg*in^2  BasedOnType=Density  Density=1000  DensityUnits=kg/(m^3)  DoExposeReferenceFrame=on  SerializedFrames=<Frames/>  GraphicType=FromGeometry  MarkerShape=Sphere  MarkerSize=10  MarkerSizeUnits=m  GraphicVisPropType=SimpleVisualProperties  GraphicDiffuseColor=[0.792157 0.819608 0.933333]  GraphicSpecularColor=[0.5 0.5 0.5 1.0]  GraphicAmbientColor=[0.15 0.15 0.15 1.0]  GraphicEmissiveColor=[0.0 0.0 0.0 1.0]  GraphicShininess=75  GraphicOpacity=1  GeometryShape=FromFile  RectangleSize=[1 1]  RectangleSizeUnits=m  BrickDimensions=[1 1 1]  BrickDimensionUnits=m  CylinderRadius=1  CylinderRadiusUnits=m  CylinderLength=1  CylinderLengthUnits=m  SphereRadius=1  SphereRadiusUnits=m  EllipsoidRadii=[1 1 1]  EllipsoidRadiiUnits=m  ExtrusionCrossSection=[1 1; -1 1; -1 -1; 1 -1]  ExtrusionCrossSectionUnits=m  ExtrusionLength=1  ExtrusionLengthUnits=m  PolygonNumSides=3  PolygonOuterRadius=1  PolygonOuterRadiusUnits=m  ExtGeomFileType=STL  ExtGeomFileName=GEAR_Default_sldprt.STL  ExtGeomFileUnits=in  RevolutionCrossSection=[1 1; 1 -1; 2 -1; 2 1]  RevolutionCrossSectionUnits=m  RevolutionExtent=Full  RevolutionAngle=180  RevolutionAngleUnits=deg
  F : PMIOPort  Side=Left
  connections:
  F/RConn1 -- ReferenceFrame/RConn1 -- Solid/RConn1

== system Quadrotor_Controller/Quadrotor Mechanics/ASSY_ROTOR_END_3_RIGID/MOTOR_1_RIGID ==
  ReferenceFrame : sm_lib/Frames and Transforms/Reference Frame
  Solid : sm_lib/Body Elements/Solid  InertiaType=Custom  Mass=0.0011134299999999999  MassUnits=kg  CenterOfMass=[0 0 -0.39208425196850388]  CenterOfMassUnits=in  MomentsOfInertia=[6.765593031186059e-05 6.765593031186059e-05 1.5113894227788452e-05]  MomentsOfInertiaUnits=kg*in^2  ProductsOfInertia=[0 0 0]  ProductsOfInertiaUnits=kg*in^2  BasedOnType=Density  Density=1000  DensityUnits=kg/(m^3)  DoExposeReferenceFrame=on  SerializedFrames=<Frames/>  GraphicType=FromGeometry  MarkerShape=Sphere  MarkerSize=10  MarkerSizeUnits=m  GraphicVisPropType=SimpleVisualProperties  GraphicDiffuseColor=[0.792157 0.819608 0.933333]  GraphicSpecularColor=[0.5 0.5 0.5 1.0]  GraphicAmbientColor=[0.15 0.15 0.15 1.0]  GraphicEmissiveColor=[0.0 0.0 0.0 1.0]  GraphicShininess=75  GraphicOpacity=1  GeometryShape=FromFile  RectangleSize=[1 1]  RectangleSizeUnits=m  BrickDimensions=[1 1 1]  BrickDimensionUnits=m  CylinderRadius=1  CylinderRadiusUnits=m  CylinderLength=1  CylinderLengthUnits=m  SphereRadius=1  SphereRadiusUnits=m  EllipsoidRadii=[1 1 1]  EllipsoidRadiiUnits=m  ExtrusionCrossSection=[1 1; -1 1; -1 -1; 1 -1]  ExtrusionCrossSectionUnits=m  ExtrusionLength=1  ExtrusionLengthUnits=m  PolygonNumSides=3  PolygonOuterRadius=1  PolygonOuterRadiusUnits=m  ExtGeomFileType=STL  ExtGeomFileName=MOTOR_Default_sldprt.STL  ExtGeomFileUnits=in  RevolutionCrossSection=[1 1; 1 -1; 2 -1; 2 1]  RevolutionCrossSectionUnits=m  RevolutionExtent=Full  RevolutionAngle=180  RevolutionAngleUnits=deg
  F : PMIOPort  Side=Left
  connections:
  F/RConn1 -- ReferenceFrame/RConn1 -- Solid/RConn1

== system Quadrotor_Controller/Quadrotor Mechanics/ASSY_ROTOR_END_3_RIGID/ROTOR_1_RIGID ==
  ReferenceFrame : sm_lib/Frames and Transforms/Reference Frame
  Solid : sm_lib/Body Elements/Solid  InertiaType=Custom  Mass=0.00139186  MassUnits=kg  CenterOfMass=[-3.0265944881889758e-07 -1.0311377952755904e-07 0.46932283464566926]  CenterOfMassUnits=in  MomentsOfInertia=[4.152148304296607e-05 0.0024363103726207443 0.0024351323702647395]  MomentsOfInertiaUnits=kg*in^2  ProductsOfInertia=[-1.4486886973773942e-11 3.7024769049538088e-11 -4.6396242792485567e-05]  ProductsOfInertiaUnits=kg*in^2  BasedOnType=Density  Density=1000  DensityUnits=kg/(m^3)  DoExposeReferenceFrame=on  SerializedFrames=<Frames/>  GraphicType=FromGeometry  MarkerShape=Sphere  MarkerSize=10  MarkerSizeUnits=m  GraphicVisPropType=SimpleVisualProperties  GraphicDiffuseColor=[0.792157 0.819608 0.933333]  GraphicSpecularColor=[0.5 0.5 0.5 1.0]  GraphicAmbientColor=[0.15 0.15 0.15 1.0]  GraphicEmissiveColor=[0.0 0.0 0.0 1.0]  GraphicShininess=75  GraphicOpacity=1  GeometryShape=FromFile  RectangleSize=[1 1]  RectangleSizeUnits=m  BrickDimensions=[1 1 1]  BrickDimensionUnits=m  CylinderRadius=1  CylinderRadiusUnits=m  CylinderLength=1  CylinderLengthUnits=m  SphereRadius=1  SphereRadiusUnits=m  EllipsoidRadii=[1 1 1]  EllipsoidRadiiUnits=m  ExtrusionCrossSection=[1 1; -1 1; -1 -1; 1 -1]  ExtrusionCrossSectionUnits=m  ExtrusionLength=1  ExtrusionLengthUnits=m  PolygonNumSides=3  PolygonOuterRadius=1  PolygonOuterRadiusUnits=m  ExtGeomFileType=STL  ExtGeomFileName=ROTOR_Default_sldprt.STL  ExtGeomFileUnits=in  RevolutionCrossSection=[1 1; 1 -1; 2 -1; 2 1]  RevolutionCrossSectionUnits=m  RevolutionExtent=Full  RevolutionAngle=180  RevolutionAngleUnits=deg
  F : PMIOPort  Side=Left
  connections:
  F/RConn1 -- ReferenceFrame/RConn1 -- Solid/RConn1

== system Quadrotor_Controller/Quadrotor Mechanics/ASSY_ROTOR_END_3_RIGID/SHAFT_1_RIGID ==
  ReferenceFrame : sm_lib/Frames and Transforms/Reference Frame
  Solid : sm_lib/Body Elements/Solid  InertiaType=Custom  Mass=0.00027398899999999998  MassUnits=kg  CenterOfMass=[0.75914960629921258 0 0.00073037401574803135]  CenterOfMassUnits=in  MomentsOfInertia=[4.8873147746295477e-07 5.0754386508772994e-05 5.076306652613304e-05]  MomentsOfInertiaUnits=kg*in^2  ProductsOfInertia=[0 -1.2690278380556758e-07 0]  ProductsOfInertiaUnits=kg*in^2  BasedOnType=Density  Density=1000  DensityUnits=kg/(m^3)  DoExposeReferenceFrame=on  SerializedFrames=<Frames/>  GraphicType=FromGeometry  MarkerShape=Sphere  MarkerSize=10  MarkerSizeUnits=m  GraphicVisPropType=SimpleVisualProperties  GraphicDiffuseColor=[0.792157 0.819608 0.933333]  GraphicSpecularColor=[0.5 0.5 0.5 1.0]  GraphicAmbientColor=[0.15 0.15 0.15 1.0]  GraphicEmissiveColor=[0.0 0.0 0.0 1.0]  GraphicShininess=75  GraphicOpacity=1  GeometryShape=FromFile  RectangleSize=[1 1]  RectangleSizeUnits=m  BrickDimensions=[1 1 1]  BrickDimensionUnits=m  CylinderRadius=1  CylinderRadiusUnits=m  CylinderLength=1  CylinderLengthUnits=m  SphereRadius=1  SphereRadiusUnits=m  EllipsoidRadii=[1 1 1]  EllipsoidRadiiUnits=m  ExtrusionCrossSection=[1 1; -1 1; -1 -1; 1 -1]  ExtrusionCrossSectionUnits=m  ExtrusionLength=1  ExtrusionLengthUnits=m  PolygonNumSides=3  PolygonOuterRadius=1  PolygonOuterRadiusUnits=m  ExtGeomFileType=STL  ExtGeomFileName=SHAFT_Default_sldprt.STL  ExtGeomFileUnits=in  RevolutionCrossSection=[1 1; 1 -1; 2 -1; 2 1]  RevolutionCrossSectionUnits=m  RevolutionExtent=Full  RevolutionAngle=180  RevolutionAngleUnits=deg
  F : PMIOPort  Side=Left
  connections:
  F/RConn1 -- ReferenceFrame/RConn1 -- Solid/RConn1

== system Quadrotor_Controller/Quadrotor Mechanics/ASSY_ROTOR_END_3_RIGID/TUBE_1_RIGID ==
  ReferenceFrame : sm_lib/Frames and Transforms/Reference Frame
  Solid : sm_lib/Body Elements/Solid  InertiaType=Custom  Mass=0.00058215999999999997  MassUnits=kg  CenterOfMass=[1.6249999999999998 0 0]  CenterOfMassUnits=in  MomentsOfInertia=[1.6501023002045999e-06 0.00051324787649575281 0.00051324787649575281]  MomentsOfInertiaUnits=kg*in^2  ProductsOfInertia=[0 0 0]  ProductsOfInertiaUnits=kg*in^2  BasedOnType=Density  Density=1000  DensityUnits=kg/(m^3)  DoExposeReferenceFrame=on  SerializedFrames=<Frames/>  GraphicType=FromGeometry  MarkerShape=Sphere  MarkerSize=10  MarkerSizeUnits=m  GraphicVisPropType=SimpleVisualProperties  GraphicDiffuseColor=[0.792157 0.819608 0.933333]  GraphicSpecularColor=[0.5 0.5 0.5 1.0]  GraphicAmbientColor=[0.15 0.15 0.15 1.0]  GraphicEmissiveColor=[0.0 0.0 0.0 1.0]  GraphicShininess=75  GraphicOpacity=1  GeometryShape=FromFile  RectangleSize=[1 1]  RectangleSizeUnits=m  BrickDimensions=[1 1 1]  BrickDimensionUnits=m  CylinderRadius=1  CylinderRadiusUnits=m  CylinderLength=1  CylinderLengthUnits=m  SphereRadius=1  SphereRadiusUnits=m  EllipsoidRadii=[1 1 1]  EllipsoidRadiiUnits=m  ExtrusionCrossSection=[1 1; -1 1; -1 -1; 1 -1]  ExtrusionCrossSectionUnits=m  ExtrusionLength=1  ExtrusionLengthUnits=m  PolygonNumSides=3  PolygonOuterRadius=1  PolygonOuterRadiusUnits=m  ExtGeomFileType=STL  ExtGeomFileName=TUBE_Default_sldprt.STL  ExtGeomFileUnits=in  RevolutionCrossSection=[1 1; 1 -1; 2 -1; 2 1]  RevolutionCrossSectionUnits=m  RevolutionExtent=Full  RevolutionAngle=180  RevolutionAngleUnits=deg
  F : PMIOPort  Side=Left
  connections:
  F/RConn1 -- ReferenceFrame/RConn1 -- Solid/RConn1

== system Quadrotor_Controller/Quadrotor Mechanics/ASSY_ROTOR_END_3_RIGID/TUBE_END_1_RIGID ==
  ReferenceFrame : sm_lib/Frames and Transforms/Reference Frame
  Solid : sm_lib/Body Elements/Solid  InertiaType=Custom  Mass=0.0014182299999999999  MassUnits=kg  CenterOfMass=[-0.0069902755905511807 -0.030264921259842512 0.077340944881889764]  CenterOfMassUnits=in  MomentsOfInertia=[0.00018641422282844559 0.00010295260090520178 0.00012412114824229644]  MomentsOfInertiaUnits=kg*in^2  ProductsOfInertia=[-4.6923243846487677e-05 7.0815766631533238e-07 1.3636989273978543e-06]  ProductsOfInertiaUnits=kg*in^2  BasedOnType=Density  Density=1000  DensityUnits=kg/(m^3)  DoExposeReferenceFrame=on  SerializedFrames=<Frames/>  GraphicType=FromGeometry  MarkerShape=Sphere  MarkerSize=10  MarkerSizeUnits=m  GraphicVisPropType=SimpleVisualProperties  GraphicDiffuseColor=[0.792157 0.819608 0.933333]  GraphicSpecularColor=[0.5 0.5 0.5 1.0]  GraphicAmbientColor=[0.15 0.15 0.15 1.0]  GraphicEmissiveColor=[0.0 0.0 0.0 1.0]  GraphicShininess=75  GraphicOpacity=1  GeometryShape=FromFile  RectangleSize=[1 1]  RectangleSizeUnits=m  BrickDimensions=[1 1 1]  BrickDimensionUnits=m  CylinderRadius=1  CylinderRadiusUnits=m  CylinderLength=1  CylinderLengthUnits=m  SphereRadius=1  SphereRadiusUnits=m  EllipsoidRadii=[1 1 1]  EllipsoidRadiiUnits=m  ExtrusionCrossSection=[1 1; -1 1; -1 -1; 1 -1]  ExtrusionCrossSectionUnits=m  ExtrusionLength=1  ExtrusionLengthUnits=m  PolygonNumSides=3  PolygonOuterRadius=1  PolygonOuterRadiusUnits=m  ExtGeomFileType=STL  ExtGeomFileName=TUBE END_Default_sldprt.STL  ExtGeomFileUnits=in  RevolutionCrossSection=[1 1; 1 -1; 2 -1; 2 1]  RevolutionCrossSectionUnits=m  RevolutionExtent=Full  RevolutionAngle=180  RevolutionAngleUnits=deg
  F : PMIOPort  Side=Left
  connections:
  F/RConn1 -- ReferenceFrame/RConn1 -- Solid/RConn1
